simulink model "PID_antiwidup"  (R2025b)
settings: Solver=ode3  StartTime=0.0  StopTime=20.0  FixedStep=1e-4  RelTol=1e-3
libraries: fillib x1
settings Model: Creator=llillo  LastModifiedBy=llillo

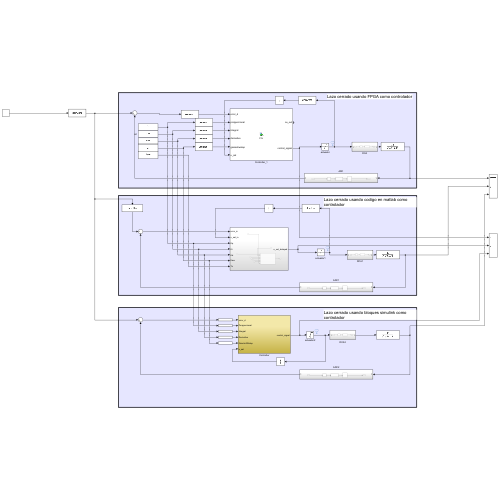
[thumbnail: Simulink's stored preview of the top-level diagram]
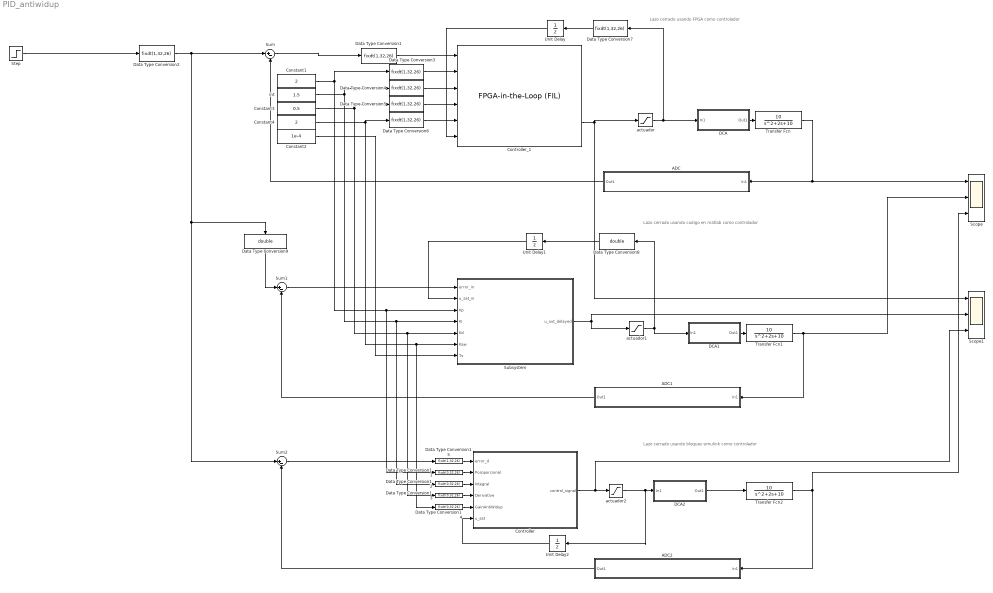
== system PID_antiwidup ==
  note: Lazo cerrado usando FPGA como controlador
  note: Lazo cerrado usando codigo en matlab como controlador
  note: Lazo cerrado usando bloques simulink como controlador
  ADC : Subsystem
  ADC1 : Subsystem
  ADC2 : Subsystem
  Constant1 : Constant  Value=2  OutDataTypeStr=double  SampleTime=1e-4  LockScale=on
  Constant2 : Constant  Value=1e-4  OutDataTypeStr=double  SampleTime=1e-4
  Constant3 : Constant  Value=0.5  OutDataTypeStr=double  SampleTime=1e-4
  Constant4 : Constant  Value=2  OutDataTypeStr=double  SampleTime=1e-4
  Controller : Subsystem  MinMaxOverflowLogging=MinMaxAndOverflow
  Controller_1 : fillib/FPGA-in-the-Loop (FIL)  ForceInterfaceUpdate=0.91338
  DCA : Subsystem
  DCA1 : Subsystem
  DCA2 : Subsystem
  Data Type Conversion{1..7,15} (8 alike) : DataTypeConversion  OutDataTypeStr=fixdt(1,32,26)  SaturateOnIntegerOverflow=off  RndMeth=Floor
  Data Type Conversion{11..14} (4 alike) : DataTypeConversion  OutDataTypeStr=fixdt(0,32,26)  SaturateOnIntegerOverflow=off  RndMeth=Floor
  Data Type Conversion8 : DataTypeConversion  OutDataTypeStr=double  SaturateOnIntegerOverflow=off  RndMeth=Floor
  Data Type Conversion9 : DataTypeConversion  OutDataTypeStr=double  SaturateOnIntegerOverflow=off  RndMeth=Floor
  Scope : Scope  NumInputPorts=3
      settings: ActiveDisplayYMinimum=-1.2274311765794395  ActiveDisplayYMaximum=11.046880589214958
  Scope1 : Scope  NumInputPorts=3
      settings: ActiveDisplayYMinimum=-1.7510604858398433  ActiveDisplayYMaximum=15.759544372558594
  Step : Step  Time=2  After=7  SampleTime=1e-4
  Subsystem : Subsystem
  Sum : Sum  Inputs=|+-
  Sum1 : Sum  Inputs=|+-
  Sum2 : Sum  Inputs=|+-
  Transfer Fcn : TransferFcn  Numerator=[10]  Denominator=[1 2 10]
  Transfer Fcn1 : TransferFcn  Numerator=[10]  Denominator=[1 2 10]
  Transfer Fcn2 : TransferFcn  Numerator=[10]  Denominator=[1 2 10]
  Unit Delay : UnitDelay  SampleTime=1e-4  HasFrameUpgradeWarning=on
  Unit Delay1 : UnitDelay  SampleTime=1e-4  HasFrameUpgradeWarning=on
  Unit Delay2 : UnitDelay  SampleTime=1e-4  HasFrameUpgradeWarning=on
  actuador : Saturate  UpperLimit=10  LowerLimit=-10  OutDataTypeStr=fixdt(1,22,16)
  actuador1 : Saturate  UpperLimit=10  LowerLimit=-10  OutDataTypeStr=fixdt(1,22,16)
  actuador2 : Saturate  UpperLimit=10  LowerLimit=-10  OutDataTypeStr=fixdt(1,32,26)
  int : Constant  Value=1.5  OutDataTypeStr=double  SampleTime=1e-4
  wires:
  ADC/1(Out1) -> Sum/2
  Transfer Fcn/1 -> ADC/1(In1), Scope/1
  DCA/1(Out1) -> Transfer Fcn/1
  actuador/1 -> Data Type Conversion7/1, DCA/1(In1)
  Step/1 -> Data Type Conversion2/1
  Data Type Conversion2/1 -> Sum/1, Sum2/1, Data Type Conversion9/1
  Sum/1 -> Data Type Conversion1/1
  Constant4/1 -> Subsystem/6(Kaw), Data Type Conversion14/1, Data Type Conversion6/1
  Constant1/1 -> Subsystem/3(Kp), Data Type Conversion11/1, Data Type Conversion3/1
  int/1 -> Subsystem/4(Ki), Data Type Conversion12/1, Data Type Conversion4/1
  Constant3/1 -> Subsystem/5(Kd), Data Type Conversion13/1, Data Type Conversion5/1
  Data Type Conversion1/1 -> Controller_1/1
  Data Type Conversion3/1 -> Controller_1/2
  Data Type Conversion4/1 -> Controller_1/3
  Data Type Conversion5/1 -> Controller_1/4
  Data Type Conversion6/1 -> Controller_1/5
  Controller_1/2 -> Scope1/1, actuador/1
  Constant2/1 -> Subsystem/7(Ts)
  Data Type Conversion7/1 -> Unit Delay/1
  Unit Delay/1 -> Controller_1/6
  Data Type Conversion8/1 -> Unit Delay1/1
  DCA1/1(Out1) -> Transfer Fcn1/1
  Transfer Fcn1/1 -> ADC1/1(In1), Scope/2
  ADC1/1(Out1) -> Sum1/2
  actuador1/1 -> DCA1/1(In1), Data Type Conversion8/1
  Data Type Conversion9/1 -> Sum1/1
  DCA2/1(Out1) -> Transfer Fcn2/1
  Controller/1(control_signal) -> Scope1/3, actuador2/1
  actuador2/1 -> Unit Delay2/1, DCA2/1(In1)
  Transfer Fcn2/1 -> Scope/3, ADC2/1(In1)
  ADC2/1(Out1) -> Sum2/2
  Sum2/1 -> Data Type Conversion15/1
  Data Type Conversion11/1 -> Controller/2(Porpporcional)
  Data Type Conversion12/1 -> Controller/3(Integral)
  Data Type Conversion13/1 -> Controller/4(Derivative)
  Data Type Conversion14/1 -> Controller/5(GainAntiWidup)
  Data Type Conversion15/1 -> Controller/1(error_d)
  Unit Delay2/1 -> Controller/6(u_sat)
  Subsystem/1(u_out_delayed) -> Scope1/2, actuador1/1
  Sum1/1 -> Subsystem/1(error_in)
  Unit Delay1/1 -> Subsystem/2(u_sat_in)

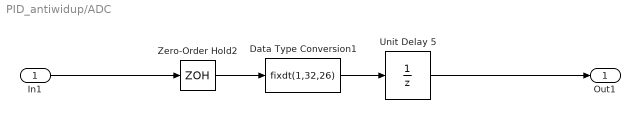
== system PID_antiwidup/ADC ==
  In1 : Inport
  Data Type Conversion1 : DataTypeConversion  OutDataTypeStr=fixdt(1,32,26)  SaturateOnIntegerOverflow=off  RndMeth=Floor
  Unit Delay 5 : UnitDelay  SampleTime=1e-4  HasFrameUpgradeWarning=on
  Zero-Order Hold2 : ZeroOrderHold  SampleTime=1e-4
  Out1 : Outport
  wires:
  Data Type Conversion1/1 -> Unit Delay 5/1
  Zero-Order Hold2/1 -> Data Type Conversion1/1
  In1/1 -> Zero-Order Hold2/1
  Unit Delay 5/1 -> Out1/1

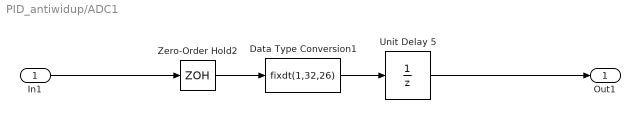
== system PID_antiwidup/ADC1 ==
  In1 : Inport
  Data Type Conversion1 : DataTypeConversion  OutDataTypeStr=fixdt(1,32,26)  SaturateOnIntegerOverflow=off  RndMeth=Floor
  Unit Delay 5 : UnitDelay  SampleTime=1e-4  HasFrameUpgradeWarning=on
  Zero-Order Hold2 : ZeroOrderHold  SampleTime=1e-4
  Out1 : Outport
  wires:
  Data Type Conversion1/1 -> Unit Delay 5/1
  Zero-Order Hold2/1 -> Data Type Conversion1/1
  In1/1 -> Zero-Order Hold2/1
  Unit Delay 5/1 -> Out1/1

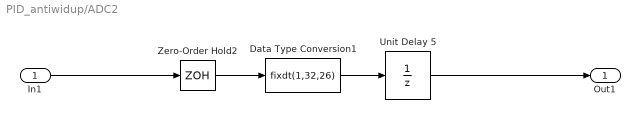
== system PID_antiwidup/ADC2 ==
  In1 : Inport
  Data Type Conversion1 : DataTypeConversion  OutDataTypeStr=fixdt(1,32,26)  SaturateOnIntegerOverflow=off  RndMeth=Floor
  Unit Delay 5 : UnitDelay  SampleTime=1e-4  HasFrameUpgradeWarning=on
  Zero-Order Hold2 : ZeroOrderHold  SampleTime=1e-4
  Out1 : Outport
  wires:
  Data Type Conversion1/1 -> Unit Delay 5/1
  Zero-Order Hold2/1 -> Data Type Conversion1/1
  In1/1 -> Zero-Order Hold2/1
  Unit Delay 5/1 -> Out1/1

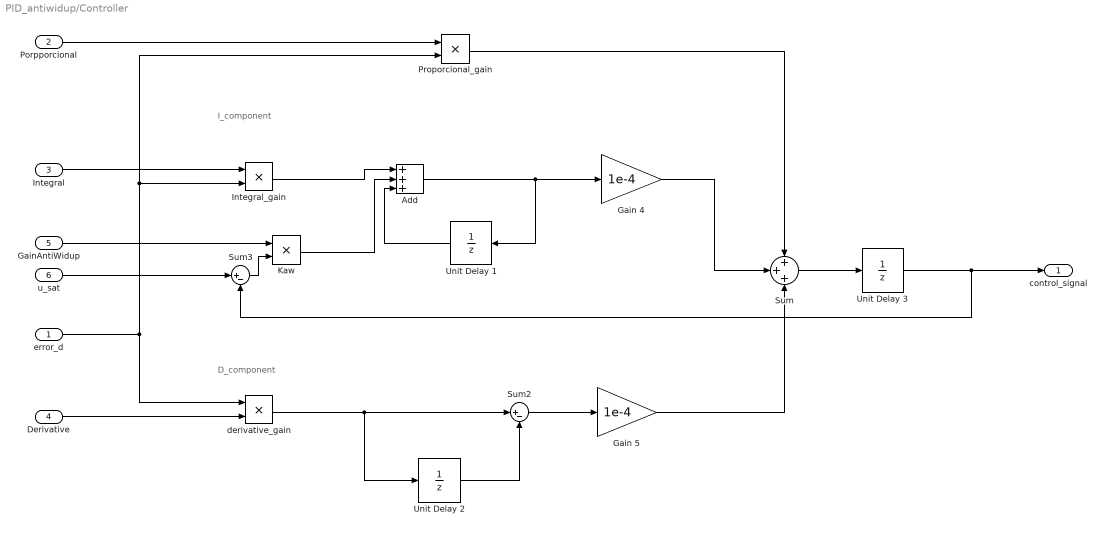
== system PID_antiwidup/Controller ==
  note: D_component
  note: I_component
  error_d : Inport  OutDataTypeStr=fixdt(1,32,26)
  Porpporcional : Inport  Port=2  OutDataTypeStr=fixdt(0,32,26)
  Integral : Inport  Port=3  OutDataTypeStr=fixdt(0,32,26)
  Derivative : Inport  Port=4  OutDataTypeStr=fixdt(0,32,26)
  GainAntiWidup : Inport  Port=5
  u_sat : Inport  Port=6
  Add : Sum  Inputs=+++  OutDataTypeStr=fixdt(1,64,26)  AccumDataTypeStr=fixdt(1,64,26)
  Gain 4 : Gain  Gain=1e-4  ParamDataTypeStr=fixdt(1,37,31)  OutDataTypeStr=fixdt(1,32,26)
  Gain 5 : Gain  Gain=1e-4  ParamDataTypeStr=fixdt(1,32,31)  OutDataTypeStr=fixdt(1,32,26)
  Integral_gain : Product  OutDataTypeStr=fixdt(1,32,26)
  Kaw : Product  OutDataTypeStr=fixdt(1,32,26)
  Proporcional_gain : Product  OutDataTypeStr=fixdt(1,32,26)
  Sum : Sum  Inputs=+++  OutDataTypeStr=fixdt(1,32,26)  AccumDataTypeStr=fixdt(1,32,26)
  Sum2 : Sum  Inputs=|+-  OutDataTypeStr=fixdt(1,32,26)  AccumDataTypeStr=fixdt(1,36,26)
  Sum3 : Sum  Inputs=|+-  OutDataTypeStr=fixdt(1,32,26)  AccumDataTypeStr=fixdt(1,32,26)
  Unit Delay 1 : UnitDelay  SampleTime=1e-4  HasFrameUpgradeWarning=on
  Unit Delay 2 : UnitDelay  SampleTime=1e-4  HasFrameUpgradeWarning=on
  Unit Delay 3 : UnitDelay  SampleTime=1e-4  HasFrameUpgradeWarning=on
  derivative_gain : Product  OutDataTypeStr=fixdt(1,32,26)
  control_signal : Outport
  wires:
  Proporcional_gain/1 -> Sum/1
  Gain 4/1 -> Sum/2
  Gain 5/1 -> Sum/3
  Sum/1 -> Unit Delay 3/1
  error_d/1 -> Integral_gain/2, Proporcional_gain/2, derivative_gain/1
  Unit Delay 2/1 -> Sum2/2
  Sum2/1 -> Gain 5/1
  derivative_gain/1 -> Unit Delay 2/1, Sum2/1
  Porpporcional/1 -> Proporcional_gain/1
  Integral/1 -> Integral_gain/1
  Derivative/1 -> derivative_gain/2
  Integral_gain/1 -> Add/1
  Add/1 -> Gain 4/1, Unit Delay 1/1
  Unit Delay 1/1 -> Add/3
  Sum3/1 -> Kaw/2
  u_sat/1 -> Sum3/1
  GainAntiWidup/1 -> Kaw/1
  Kaw/1 -> Add/2
  Unit Delay 3/1 -> Sum3/2, control_signal/1

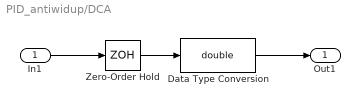
== system PID_antiwidup/DCA ==
  In1 : Inport
  Data Type Conversion : DataTypeConversion  OutDataTypeStr=double  SaturateOnIntegerOverflow=off  RndMeth=Floor
  Zero-Order Hold : ZeroOrderHold  SampleTime=1e-4
  Out1 : Outport
  wires:
  Zero-Order Hold/1 -> Data Type Conversion/1
  Data Type Conversion/1 -> Out1/1
  In1/1 -> Zero-Order Hold/1

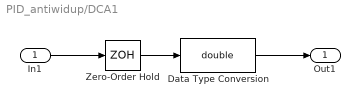
== system PID_antiwidup/DCA1 ==
  In1 : Inport
  Data Type Conversion : DataTypeConversion  OutDataTypeStr=double  SaturateOnIntegerOverflow=off  RndMeth=Floor
  Zero-Order Hold : ZeroOrderHold  SampleTime=1e-4
  Out1 : Outport
  wires:
  Zero-Order Hold/1 -> Data Type Conversion/1
  Data Type Conversion/1 -> Out1/1
  In1/1 -> Zero-Order Hold/1

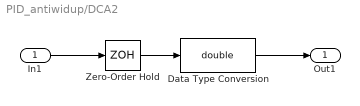
== system PID_antiwidup/DCA2 ==
  In1 : Inport
  Data Type Conversion : DataTypeConversion  OutDataTypeStr=double  SaturateOnIntegerOverflow=off  RndMeth=Floor
  Zero-Order Hold : ZeroOrderHold  SampleTime=1e-4
  Out1 : Outport
  wires:
  Zero-Order Hold/1 -> Data Type Conversion/1
  Data Type Conversion/1 -> Out1/1
  In1/1 -> Zero-Order Hold/1

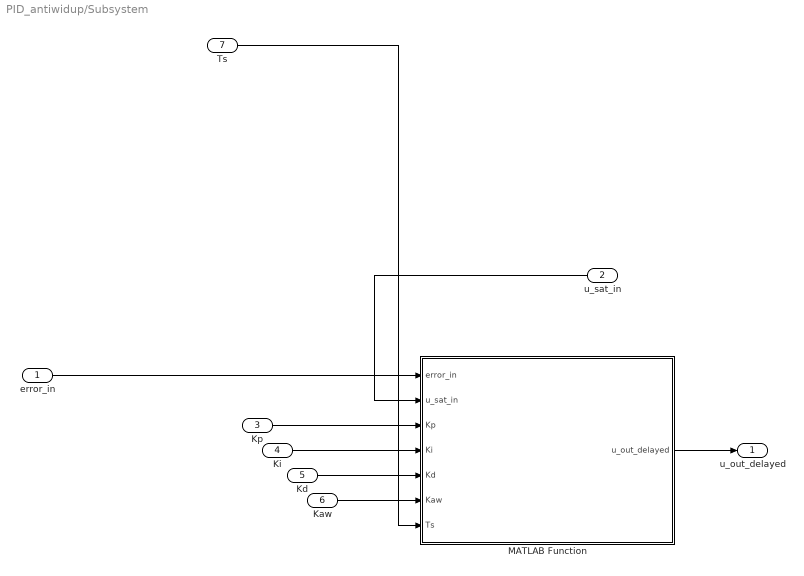
== system PID_antiwidup/Subsystem ==
  error_in : Inport
  u_sat_in : Inport  Port=2
  Kp : Inport  Port=3
  Ki : Inport  Port=4
  Kd : Inport  Port=5
  Kaw : Inport  Port=6
  Ts : Inport  Port=7
  MATLAB Function : MATLAB Function  TreatAsAtomicUnit=on
  u_out_delayed : Outport
  wires:
  Kp/1 -> MATLAB Function/3(Kp)
  error_in/1 -> MATLAB Function/1(error_in)
  MATLAB Function/1(u_out_delayed) -> u_out_delayed/1
  Kaw/1 -> MATLAB Function/6(Kaw)
  u_sat_in/1 -> MATLAB Function/2(u_sat_in)
  Ts/1 -> MATLAB Function/7(Ts)
  Kd/1 -> MATLAB Function/5(Kd)
  Ki/1 -> MATLAB Function/4(Ki)

== matlab function PID_antiwidup/Subsystem/MATLAB Function ==
  data: error_in input; u_out_delayed output; u_sat_in input; Kp input; Ki input; Kd input; Kaw input; Ts input
function u_out_delayed = PID_antiwindup(error_in, u_sat_in, Kp, Ki, Kd, Kaw, Ts)
    % el assert se usa para que la herramienta de fixed point le sea ams
    % facil entender qu es un escalar y no una matriz cada entrada
    assert(isscalar(error_in));
    assert(isscalar(u_sat_in));
    assert(isscalar(Kp));
    assert(isscalar(Ki));
    assert(isscalar(Kd));
    assert(isscalar(Kaw));
    assert(isscalar(Ts));
    % -----------------------------------------

    persistent I_prev val_prod_prev u_total_prev
    
    if isempty(I_prev)
        I_prev = 0;         
        val_prod_prev = 0;  
        u_total_prev = 0;   
    end
    
    % P
    P = Kp * error_in;
    
    % D
    val_prod_actual = Kd * error_in;
    resta_D         = val_prod_actual - val_prod_prev;
    D               = resta_D * Ts; 
    u_calc          = P + I_prev + D;
    
    % I
    diff_aw     = u_sat_in - u_calc;
    term_aw     = Kaw * diff_aw;
    term_ki     = Ki * error_in;
    suma_I      = term_ki + term_aw;
    I_increment = suma_I * Ts;
    I_new       = I_increment + I_prev;
    
    % out
    u_out_delayed = u_total_prev;
    
    % actualizar estaod anterior
    I_prev        = I_new;
    val_prod_prev = val_prod_actual;
    u_total_prev  = u_calc;
end
